simulink model "soc_rfsoc_fpga"  (R2023b)
settings: Solver=FixedStepDiscrete  StartTime=0.0  StopTime=15e-4  RelTol=1e-3  EnableMultiTasking=on
undefined symbols (not defined in the file): SampleTime
libraries: hwlogicconnlib x4
settings Model: DataTypeOverride=Off  Creator=The MathWorks, Inc.  LastModifiedBy=akroh
settings SolverCC: AlgebraicLoopSolver=TrustRegion  PositivePriorityOrder=on  MaxZcPerStep=1
settings DataIOCC: SaveOutput=off  SaveTime=off  ReturnWorkspaceOutputs=off
settings OptimizationCC: BlockReduction=off  ConditionallyExecuteInputs=off  DefaultParameterBehavior=Inlined  PassReuseOutputArgsAs=Individual arguments  MaxStackSize=64  EfficientTunableParamExpr=on
settings DebuggingCC: AlgebraicLoopMsg=error  SingleTaskRateTransMsg=error  IntegerOverflowMsg=none  ParameterPrecisionLossMsg=none  ParameterTunabilityLossMsg=error  UnconnectedInputMsg=warning  UnconnectedOutputMsg=warning  UnconnectedLineMsg=warning  PregeneratedLibrarySubsystemCodeDiagnostic=none  SFUnexpectedBacktrackingDiag=warning  SFNoUnconditionalDefaultTransitionDiag=warning  ArithmeticOperatorsInVariantConditions=warning
settings HardwareCC: ProdBitPerPointer=32  ProdBitPerSizeT=32  ProdBitPerPtrDiffT=32  ProdLargestAtomicFloat=None  ProdIntDivRoundTo=Undefined  ProdEndianess=Unspecified  ProdWordSize=32  ProdHWDeviceType=ASIC/FPGA->ASIC/FPGA  TargetBitPerLong=64  TargetBitPerPointer=64  TargetBitPerSizeT=64  TargetBitPerPtrDiffT=64  TargetLongLongMode=on  TargetIntDivRoundTo=Zero  TargetEndianess=LittleEndian  TargetWordSize=64  TargetHWDeviceType=Custom Processor->MATLAB Host Computer  ProdEqTarget=off
settings ModelReferenceCC: EnableRefExpFcnMdlSchedulingChecks=on
settings SFSimCC: SimUseLocalCustomCode=off  MATLABDynamicMemAlloc=off
settings RTWCC: Description=Embedded Coder  SystemTargetFile=ert.tlc  TemplateMakefile=ert_default_tmf  GenerateReport=on  RTWUseLocalCustomCode=off  Toolchain=Linaro AArch32 Linux v6.3.1  IncludeHyperlinkInReport=on  LaunchReport=on  GenerateTraceInfo=on  GenerateTraceReport=on  GenerateTraceReportSl=on  GenerateTraceReportSf=on  GenerateTraceReportEml=on  DLArmComputeVersion=19.05
settings CodeAppCC: ForceParamTrailComments=on  IgnoreCustomStorageClasses=off  OperatorAnnotations=on  SimulinkDataObjDesc=on  SFDataObjDesc=on  InsertBlockDesc=on
settings ERTTargetCC: ERTCustomFileTemplate=example_file_process.tlc

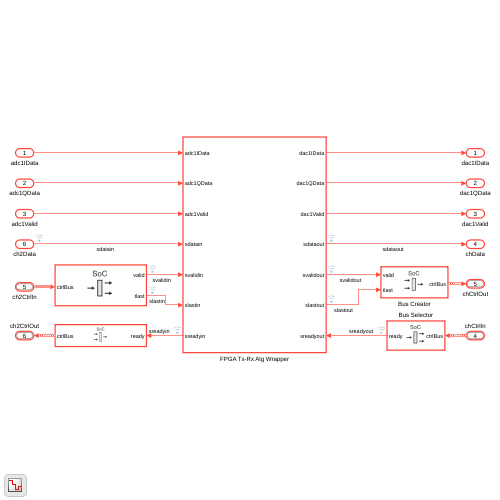
[thumbnail: Simulink's stored preview of the top-level diagram]
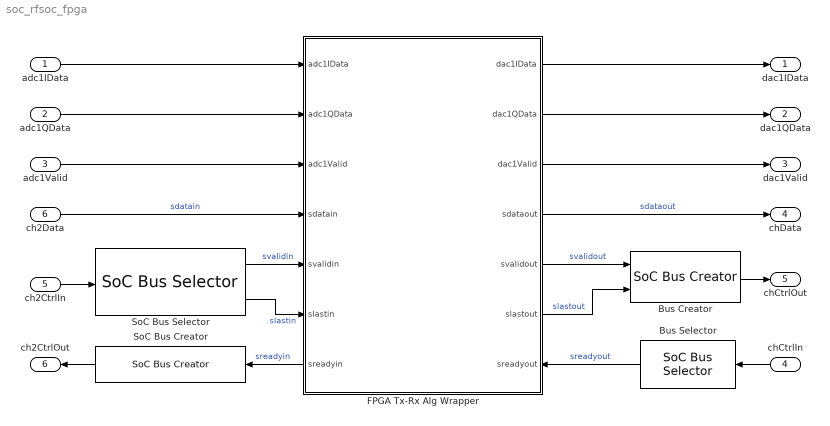
== system soc_rfsoc_fpga ==
  adc1IData : Inport  OutDataTypeStr=uint32  SampleTime=SampleTime
  adc1QData : Inport  Port=2  OutDataTypeStr=uint32
  adc1Valid : Inport  Port=3  OutDataTypeStr=boolean
  chCtrlIn : Inport  Port=4  OutDataTypeStr=Bus: StreamS2MBusObj  BusOutputAsStruct=on
  ch2CtrlIn : Inport  Port=5  OutDataTypeStr=Bus: StreamM2SBusObj
  ch2Data : Inport  Port=6  OutDataTypeStr=uint32
  Bus Creator : hwlogicconnlib/SoC Bus Creator  Protocol=Data stream  ctrltype=Valid
  Bus Selector : hwlogicconnlib/SoC Bus Selector  Protocol=Data stream  ctrltype=Ready
  FPGA Tx-Rx Alg Wrapper : Subsystem  TreatAsAtomicUnit=on
      settings: PortSchema="{\"entries\":[{\"content\":{\"sides\":[{\"content\":{\"connectorIds\":[\"In1\",\"In2\",\"In3\",\"In4\",\"In5\",\"In6\",\"Out7\"]},\"type\":\"ConnectorPlacement.EquallySpacedRectSide\",\"uuid\":\"ace61bd0-2bb3-4c57-8405-0a69ae17f2d0\"},{\"content\":{\"connectorIds\":[\"Out1\",\"Out2\",\"Out3\",\"Out4\",\"Out5\",\"Out6\",\"In7\"],\"side\":\"RIGHT\"},\"type\":\"ConnectorPlacement.EquallySpacedRectSide\",\"uuid\":\"2e0d9ccd-a935-4706-bed3-fe39e394506e\"},{\"content\":{\"side\":\"TOP\"},\"type\":\"ConnectorPlacement.EquallySpacedRectSide\",\"uuid\":\"d64ee626-d3ec-4a41-b8a5-0770f1865b04\"}]},\"type\":\"ConnectorPlacement.EquallySpacedConnector\",\"uuid\":\"515a1d06-9e93-401b-b672-970be835262d\"}],\"packageUris\":[\"http://schema.mathworks.com/mf0/Connector/R2020b\"],\"version\":\"1.0\"}"
  SoC Bus Creator : hwlogicconnlib/SoC Bus Creator  Protocol=Data stream  ctrltype=Ready
  SoC Bus Selector : hwlogicconnlib/SoC Bus Selector  Protocol=Data stream  ctrltype=Valid
  dac1IData : Outport  VectorParamsAs1DForOutWhenUnconnected=off
  dac1QData : Outport  Port=2  VectorParamsAs1DForOutWhenUnconnected=off
  dac1Valid : Outport  Port=3  VectorParamsAs1DForOutWhenUnconnected=off
  chData : Outport  Port=4  OutDataTypeStr=uint32  VectorParamsAs1DForOutWhenUnconnected=off
  chCtrlOut : Outport  Port=5  OutDataTypeStr=Bus: StreamM2SBusObj  VectorParamsAs1DForOutWhenUnconnected=off  BusOutputAsStruct=on
  ch2CtrlOut : Outport  Port=6  OutDataTypeStr=Bus: StreamS2MBusObj
  wires:
  adc1QData/1 -> FPGA Tx-Rx Alg Wrapper/2(adc1QData)
  adc1IData/1 -> FPGA Tx-Rx Alg Wrapper/1(adc1IData)
  Bus Creator/1 -> chCtrlOut/1
  chCtrlIn/1 -> Bus Selector/1
  FPGA Tx-Rx Alg Wrapper/1(dac1IData) -> dac1IData/1
  FPGA Tx-Rx Alg Wrapper/2(dac1QData) -> dac1QData/1
  FPGA Tx-Rx Alg Wrapper/3(dac1Valid) -> dac1Valid/1
  adc1Valid/1 -> FPGA Tx-Rx Alg Wrapper/3(adc1Valid)
  Bus Selector/1 -> FPGA Tx-Rx Alg Wrapper/7(sreadyout)  "sreadyout"
  FPGA Tx-Rx Alg Wrapper/5(svalidout) -> Bus Creator/1  "svalidout"
  FPGA Tx-Rx Alg Wrapper/6(slastout) -> Bus Creator/2  "slastout"
  FPGA Tx-Rx Alg Wrapper/4(sdataout) -> chData/1  "sdataout"
  SoC Bus Selector/1 -> FPGA Tx-Rx Alg Wrapper/5(svalidin)  "svalidin"
  FPGA Tx-Rx Alg Wrapper/7(sreadyin) -> SoC Bus Creator/1  "sreadyin"
  ch2CtrlIn/1 -> SoC Bus Selector/1
  SoC Bus Creator/1 -> ch2CtrlOut/1
  ch2Data/1 -> FPGA Tx-Rx Alg Wrapper/4(sdatain)  "sdatain"
  SoC Bus Selector/2 -> FPGA Tx-Rx Alg Wrapper/6(slastin)  "slastin"

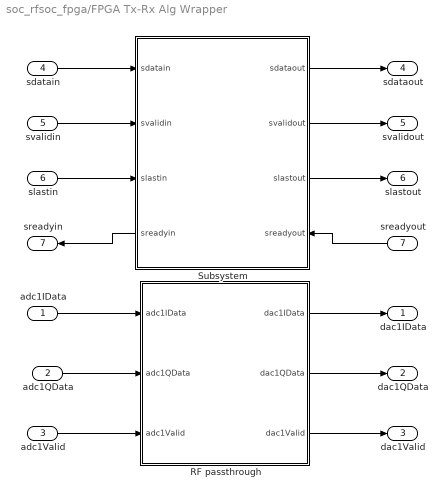
== system soc_rfsoc_fpga/FPGA Tx-Rx Alg Wrapper ==
  adc1IData : Inport
  adc1QData : Inport  Port=2
  adc1Valid : Inport  Port=3
  sdatain : Inport  Port=4
  svalidin : Inport  Port=5
  slastin : Inport  Port=6
  sreadyout : Inport  Port=7
  RF passthrough : Subsystem
  Subsystem : Subsystem
      settings: PortSchema="{\"entries\":[{\"content\":{\"sides\":[{\"content\":{\"connectorIds\":[\"In1\",\"In2\",\"In3\",\"Out4\"]},\"type\":\"ConnectorPlacement.EquallySpacedRectSide\",\"uuid\":\"42e5c2cd-e0c8-4138-8990-974bb331ef6e\"},{\"content\":{\"connectorIds\":[\"Out1\",\"Out2\",\"Out3\",\"In4\"],\"side\":\"RIGHT\"},\"type\":\"ConnectorPlacement.EquallySpacedRectSide\",\"uuid\":\"211e8ed3-40ae-4dcc-a64e-400744573b3b\"},{\"content\":{\"side\":\"TOP\"},\"type\":\"ConnectorPlacement.EquallySpacedRectSide\",\"uuid\":\"24e02230-0b01-4758-9091-d97173d39cbf\"}]},\"type\":\"ConnectorPlacement.EquallySpacedConnector\",\"uuid\":\"1b6e945e-46e4-49b4-832b-cd4b96e17652\"}],\"packageUris\":[\"http://schema.mathworks.com/mf0/Connector/R2020b\"],\"version\":\"1.0\"}"
  dac1IData : Outport  VectorParamsAs1DForOutWhenUnconnected=off
  dac1QData : Outport  Port=2  VectorParamsAs1DForOutWhenUnconnected=off
  dac1Valid : Outport  Port=3  VectorParamsAs1DForOutWhenUnconnected=off
  sdataout : Outport  Port=4
  svalidout : Outport  Port=5
  slastout : Outport  Port=6
  sreadyin : Outport  Port=7
  wires:
  sreadyout/1 -> Subsystem/4(sreadyout)
  sdatain/1 -> Subsystem/1(sdatain)
  adc1Valid/1 -> RF passthrough/3(adc1Valid)
  slastin/1 -> Subsystem/3(slastin)
  adc1IData/1 -> RF passthrough/1(adc1IData)
  Subsystem/2(svalidout) -> svalidout/1
  adc1QData/1 -> RF passthrough/2(adc1QData)
  RF passthrough/1(dac1IData) -> dac1IData/1
  Subsystem/4(sreadyin) -> sreadyin/1
  Subsystem/3(slastout) -> slastout/1
  Subsystem/1(sdataout) -> sdataout/1
  svalidin/1 -> Subsystem/2(svalidin)
  RF passthrough/2(dac1QData) -> dac1QData/1
  RF passthrough/3(dac1Valid) -> dac1Valid/1

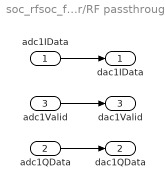
== system soc_rfsoc_fpga/FPGA Tx-Rx Alg Wrapper/RF passthrough ==
  adc1IData : Inport
  adc1QData : Inport  Port=2
  adc1Valid : Inport  Port=3
  dac1IData : Outport  VectorParamsAs1DForOutWhenUnconnected=off
  dac1QData : Outport  Port=2  VectorParamsAs1DForOutWhenUnconnected=off
  dac1Valid : Outport  Port=3  VectorParamsAs1DForOutWhenUnconnected=off
  wires:
  adc1QData/1 -> dac1QData/1
  adc1Valid/1 -> dac1Valid/1
  adc1IData/1 -> dac1IData/1

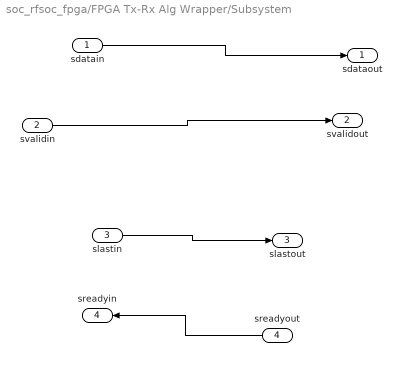
== system soc_rfsoc_fpga/FPGA Tx-Rx Alg Wrapper/Subsystem ==
  sdatain : Inport
  svalidin : Inport  Port=2
  slastin : Inport  Port=3
  sreadyout : Inport  Port=4
  sdataout : Outport
  svalidout : Outport  Port=2
  slastout : Outport  Port=3
  sreadyin : Outport  Port=4
  wires:
  svalidin/1 -> svalidout/1
  sreadyout/1 -> sreadyin/1
  sdatain/1 -> sdataout/1
  slastin/1 -> slastout/1
